simulink model "Fulladder_Model"  (R2025a)
settings: Solver=VariableStepAuto  StartTime=0.0  StopTime=10.0  RelTol=1e-3
libraries: NSA_DEVS_SINKS x5, NSA_DEVS_SOURCES x3, NSA_DEVS_LOGISTICS x2, NSA_DEVS_DIGITALI3E_LOGIC x1
settings Model: Creator=david  LastModifiedBy=peter
settings RTWCC: GPUComputeCapability=3.5

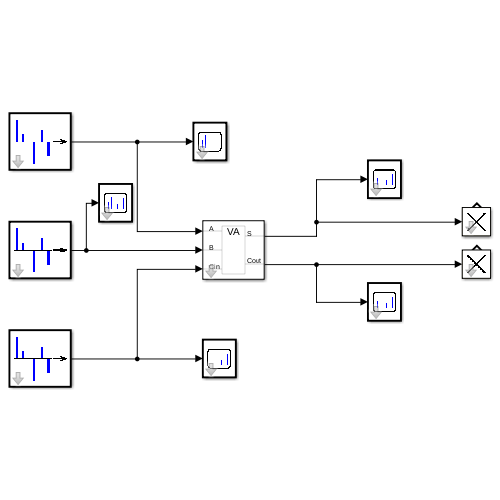
[thumbnail: Simulink's stored preview of the top-level diagram]
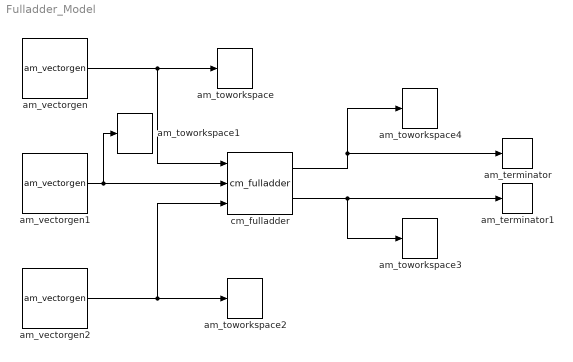
== system Fulladder_Model ==
  am_terminator : NSA_DEVS_LOGISTICS/am_terminator  tau=[0,1]  debug=0
      settings: SourceProductName=Logistics
  am_terminator1 : NSA_DEVS_LOGISTICS/am_terminator  tau=[0,1]  debug=0
      settings: SourceProductName=Logistics
  am_toworkspace : NSA_DEVS_SINKS/am_toworkspace  varname="\"gen1Out\""  t0=0  format="\"vector\""  tau=[0,5]  debug=0
      settings: SourceProductName=Sinks
  am_toworkspace1 : NSA_DEVS_SINKS/am_toworkspace  varname="\"gen2Out\""  t0=0  format="\"vector\""  tau=[0,5]  debug=0
      settings: SourceProductName=Sinks
  am_toworkspace2 : NSA_DEVS_SINKS/am_toworkspace  varname="\"gen3Out\""  t0=0  format="\"vector\""  tau=[0,5]  debug=0
      settings: SourceProductName=Sinks
  am_toworkspace3 : NSA_DEVS_SINKS/am_toworkspace  varname="\"facOut\""  t0=0  format="\"vector\""  tau=[0,5]  debug=0
      settings: SourceProductName=Sinks
  am_toworkspace4 : NSA_DEVS_SINKS/am_toworkspace  varname="\"fasOut\""  t0=0  format="\"vector\""  tau=[0,5]  debug=0
      settings: SourceProductName=Sinks
  am_vectorgen : NSA_DEVS_SOURCES/am_vectorgen  tvec=[1, 2, 3, 6, 7, 8, 9, 12]  yvec="[\"0\", \"1\", \"0\", \"1\", \"0\", \"1\", \"0\", \"1\"]"  tau=[0,1]  debug=0
      settings: SourceProductName=Sources
  am_vectorgen1 : NSA_DEVS_SOURCES/am_vectorgen  tvec=[1, 4, 5, 6, 7, 10, 11, 12]  yvec="[\"0\", \"1\", \"0\", \"1\", \"0\", \"1\",  \"0\",  \"1\"]"  tau=[0,1]  debug=0
      settings: SourceProductName=Sources
  am_vectorgen2 : NSA_DEVS_SOURCES/am_vectorgen  tvec=[1, 4, 5, 6, 7, 12]  yvec="[\"0\", \"0\", \"0\", \"0\", \"1\", \"1\"]"  tau=[0,1]  debug=0
      settings: SourceProductName=Sources
  cm_fulladder : NSA_DEVS_DIGITALI3E_LOGIC/cm_fulladder  tau=[0,1]  debug=0
  wires:
  am_vectorgen1/1 -> am_toworkspace1/1, cm_fulladder/2
  am_vectorgen/1 -> am_toworkspace/1, cm_fulladder/1
  am_vectorgen2/1 -> am_toworkspace2/1, cm_fulladder/3
  cm_fulladder/1 -> am_toworkspace4/1, am_terminator/1
  cm_fulladder/2 -> am_toworkspace3/1, am_terminator1/1
